simulink model "Code_Gen_Model"  (R2025a)
settings: Solver=FixedStepDiscrete  StartTime=0.0  StopTime=inf  FixedStep=t_sample  RelTol=1e-3
settings Model: Creator=FIRSTMentor  LastModifiedBy=ander
settings OptimizationCC: DefaultParameterBehavior=Inlined  StrengthReduction=on  PassReuseOutputArgsAs=Individual arguments  ZeroExternalMemoryAtStartup=off  ZeroInternalMemoryAtStartup=off  OptimizeBlockOrder=speed  OptimizationPriority=Speed  OptimizationCustomize=off  MultiThreadedLoops=on  AutoScheduleForLoops=on  EfficientTunableParamExpr=on
settings DebuggingCC: MergeDetectMultiDrivingBlocksExec=none  ParameterTunabilityLossMsg=error
settings HardwareCC: ProdBitPerPointer=32.0  ProdBitPerSizeT=32.0  ProdBitPerPtrDiffT=32.0  ProdLargestAtomicInteger=Long  ProdWordSize=32.0  ProdHWDeviceType=ARM Compatible->ARM 7
settings ModelReferenceCC: PropagateSignalLabelsOutOfModel=off
settings SFSimCC: MATLABDynamicMemAlloc=off
settings RTWCC: SystemTargetFile=ert.tlc  GenCodeOnly=on  TemplateMakefile=ert_default_tmf  Toolchain=MinGW64 | gmake (64-bit Windows)  GPUComputeCapability=3.5  Description=Embedded Coder
settings CodeAppCC: ForceParamTrailComments=on  IgnoreCustomStorageClasses=off  OperatorAnnotations=on  SimulinkDataObjDesc=on  SFDataObjDesc=on  InsertBlockDesc=on
settings ERTTargetCC: ExtModeTransport=0.0  ExtModeStaticAlloc=off  ExtModeMexFile=ext_comm  ExtModeIntrfLevel=Level1  ERTCustomFileTemplate=example_file_process.tlc  DynamicArrayContainerType=coder::array  TargetLangStandard=C99 (ISO)  SupportVariableSizeSignals=on  ParenthesesLevel=Maximum

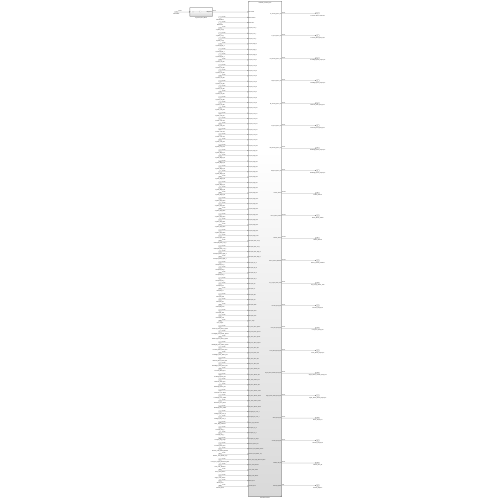
[thumbnail: Simulink's stored preview of the top-level diagram]
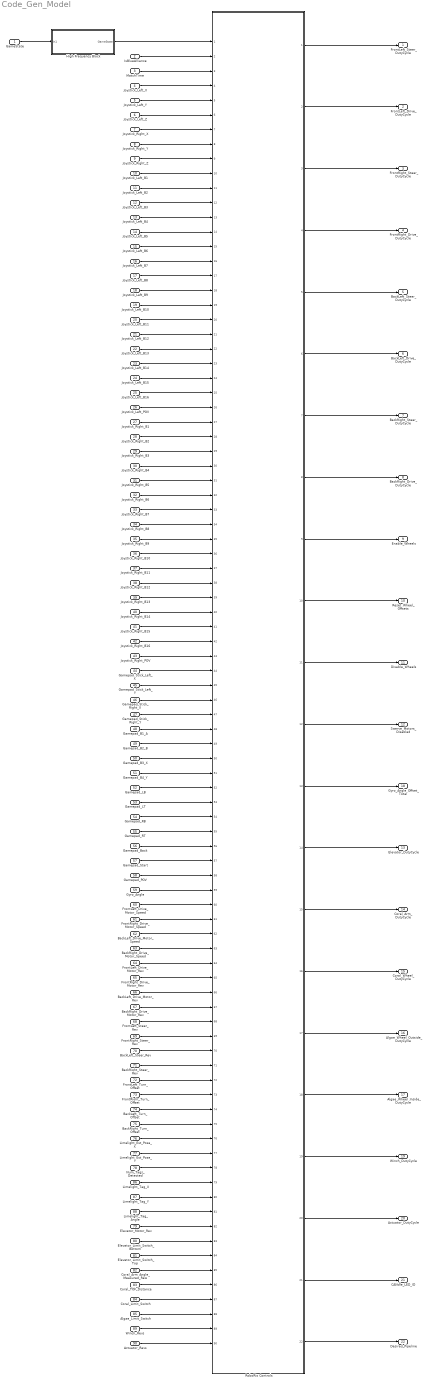
== system Code_Gen_Model ==
  GameState : Inport
  IsBlueAlliance : Inport  Port=2
  MatchTime : Inport  Port=3
  Joystick_Left_X : Inport  Port=4
  Joystick_Left_Y : Inport  Port=5
  Joystick_Left_Z : Inport  Port=6
  Joystick_Right_X : Inport  Port=7
  Joystick_Right_Y : Inport  Port=8
  Joystick_Right_Z : Inport  Port=9
  Joystick_Left_B1 : Inport  Port=10
  Joystick_Left_B2 : Inport  Port=11
  Joystick_Left_B3 : Inport  Port=12
  Joystick_Left_B4 : Inport  Port=13
  Joystick_Left_B5 : Inport  Port=14
  Joystick_Left_B6 : Inport  Port=15
  Joystick_Left_B7 : Inport  Port=16
  Joystick_Left_B8 : Inport  Port=17
  Joystick_Left_B9 : Inport  Port=18
  Joystick_Left_B10 : Inport  Port=19
  Joystick_Left_B11 : Inport  Port=20
  Joystick_Left_B12 : Inport  Port=21
  Joystick_Left_B13 : Inport  Port=22
  Joystick_Left_B14 : Inport  Port=23
  Joystick_Left_B15 : Inport  Port=24
  Joystick_Left_B16 : Inport  Port=25
  Joystick_Left_POV : Inport  Port=26
  Joystick_Right_B1 : Inport  Port=27
  Joystick_Right_B2 : Inport  Port=28
  Joystick_Right_B3 : Inport  Port=29
  Joystick_Right_B4 : Inport  Port=30
  Joystick_Right_B5 : Inport  Port=31
  Joystick_Right_B6 : Inport  Port=32
  Joystick_Right_B7 : Inport  Port=33
  Joystick_Right_B8 : Inport  Port=34
  Joystick_Right_B9 : Inport  Port=35
  Joystick_Right_B10 : Inport  Port=36
  Joystick_Right_B11 : Inport  Port=37
  Joystick_Right_B12 : Inport  Port=38
  Joystick_Right_B13 : Inport  Port=39
  Joystick_Right_B14 : Inport  Port=40
  Joystick_Right_B15 : Inport  Port=41
  Joystick_Right_B16 : Inport  Port=42
  Joystick_Right_POV : Inport  Port=43
  Gamepad_Stick_Left_X : Inport  Port=44
  Gamepad_Stick_Left_Y : Inport  Port=45
  Gamepad_Stick_Right_X : Inport  Port=46
  Gamepad_Stick_Right_Y : Inport  Port=47
  Gamepad_B1_A : Inport  Port=48
  Gamepad_B2_B : Inport  Port=49
  Gamepad_B3_X : Inport  Port=50
  Gamepad_B4_Y : Inport  Port=51
  Gamepad_LB : Inport  Port=52
  Gamepad_LT : Inport  Port=53
  Gamepad_RB : Inport  Port=54
  Gamepad_RT : Inport  Port=55
  Gamepad_Back : Inport  Port=56
  Gamepad_Start : Inport  Port=57
  Gamepad_POV : Inport  Port=58
  Gyro_Angle : Inport  Port=59
  FrontLeft_Drive_Motor_Speed : Inport  Port=60
  FrontRight_Drive_Motor_Speed : Inport  Port=61
  BackLeft_Drive_Motor_Speed : Inport  Port=62
  BackRight_Drive_Motor_Speed : Inport  Port=63
  FrontLeft_Drive_Motor_Rev : Inport  Port=64
  FrontRight_Drive_Motor_Rev : Inport  Port=65
  BackLeft_Drive_Motor_Rev : Inport  Port=66
  BackRight_Drive_Motor_Rev : Inport  Port=67
  FrontLeft_Steer_Rev : Inport  Port=68
  FrontRight_Steer_Rev : Inport  Port=69
  BackLeft_Steer_Rev : Inport  Port=70
  BackRight_Steer_Rev : Inport  Port=71
  FrontLeft_Turn_Offset : Inport  Port=72
  FrontRight_Turn_Offset : Inport  Port=73
  BackLeft_Turn_Offset : Inport  Port=74
  BackRight_Turn_Offset : Inport  Port=75
  Limelight_Est_Pose_X : Inport  Port=76
  Limelight_Est_Pose_Y : Inport  Port=77
  Num_Tags_Detected : Inport  Port=78
  Elevator_Motor_Rev : Inport  Port=79
  Elevator_Limit_Switch_Bottom : Inport  Port=80
  Elevator_Limit_Switch_Top : Inport  Port=81
  Coral_Arm_Angle_Measured_Raw : Inport  Port=82
  Coral_TOF_Distance : Inport  Port=83
  Coral_Limit_Switch : Inport  Port=84
  Algae_Limit_Switch : Inport  Port=85
  Limelight_Tag_X : Inport  Port=86
  Limelight_Tag_Y : Inport  Port=87
  Limelight_Tag_Angle : Inport  Port=88
  Winch_Revs : Inport  Port=89
  Actuator_Revs : Inport  Port=90
  High Frequency Block : Subsystem  TreatAsAtomicUnit=on  RTWFcnName=High_Frequency_Model_Step
      settings: RTWSystemCode=Nonreusable function  RTWFcnNameOpts=User specified
  RoboRio Controls : Subsystem  TreatAsAtomicUnit=on  RTWFcnName=Model_Step  ReferencedSubsystem=RoboRio_Controls_sub
      settings: RTWSystemCode=Nonreusable function  RTWFcnNameOpts=User specified
  FrontLeft_Steer_DutyCycle : Outport
  FrontLeft_Drive_DutyCycle : Outport  Port=2
  FrontRight_Steer_DutyCycle : Outport  Port=3
  FrontRight_Drive_DutyCycle : Outport  Port=4
  BackLeft_Steer_DutyCycle : Outport  Port=5
  BackLeft_Drive_DutyCycle : Outport  Port=6
  BackRight_Steer_DutyCycle : Outport  Port=7
  BackRight_Drive_DutyCycle : Outport  Port=8
  Enable_Wheels : Outport  Port=9
  Reset_Wheel_Offsets : Outport  Port=10
  Disable_Wheels : Outport  Port=11
  Swerve_Motors_Disabled : Outport  Port=12
  Elevator_DutyCycle : Outport  Port=13
  Coral_Arm_DutyCycle : Outport  Port=14
  Coral_Wheel_DutyCycle : Outport  Port=15
  Algae_Wheel_Outside_DutyCycle : Outport  Port=16
  Algae_Wheel_Inside_DutyCycle : Outport  Port=17
  Gyro_Angle_Offset_Total : Outport  Port=18
  Winch_DutyCycle : Outport  Port=19
  Actuator_DutyCycle : Outport  Port=20
  CANdle_LED_ID : Outport  Port=21
  Desired_Pipeline : Outport  Port=22
  wires:
  Joystick_Right_B10/1 -> RoboRio Controls/36
  Joystick_Right_B8/1 -> RoboRio Controls/34
  Joystick_Right_B7/1 -> RoboRio Controls/33
  Joystick_Right_B4/1 -> RoboRio Controls/30
  High Frequency Block/1(GameState) -> RoboRio Controls/1
  RoboRio Controls/8 -> BackRight_Drive_DutyCycle/1
  Gamepad_Stick_Left_X/1 -> RoboRio Controls/44
  Joystick_Right_POV/1 -> RoboRio Controls/43
  Joystick_Right_B14/1 -> RoboRio Controls/40
  Joystick_Right_B13/1 -> RoboRio Controls/39
  Joystick_Right_B3/1 -> RoboRio Controls/29
  Joystick_Right_B2/1 -> RoboRio Controls/28
  Joystick_Right_B1/1 -> RoboRio Controls/27
  Joystick_Left_POV/1 -> RoboRio Controls/26
  Limelight_Est_Pose_Y/1 -> RoboRio Controls/77
  Joystick_Left_Z/1 -> RoboRio Controls/6
  Joystick_Left_Y/1 -> RoboRio Controls/5
  Joystick_Left_X/1 -> RoboRio Controls/4
  IsBlueAlliance/1 -> RoboRio Controls/2
  Gamepad_B2_B/1 -> RoboRio Controls/49
  Joystick_Left_B1/1 -> RoboRio Controls/10
  Joystick_Right_Z/1 -> RoboRio Controls/9
  RoboRio Controls/3 -> FrontRight_Steer_DutyCycle/1
  Joystick_Right_Y/1 -> RoboRio Controls/8
  Joystick_Right_X/1 -> RoboRio Controls/7
  BackRight_Steer_Rev/1 -> RoboRio Controls/71
  Joystick_Left_B7/1 -> RoboRio Controls/16
  FrontRight_Steer_Rev/1 -> RoboRio Controls/69
  Joystick_Left_B4/1 -> RoboRio Controls/13
  Joystick_Left_B3/1 -> RoboRio Controls/12
  Joystick_Left_B2/1 -> RoboRio Controls/11
  Joystick_Left_B14/1 -> RoboRio Controls/23
  Joystick_Left_B13/1 -> RoboRio Controls/22
  Joystick_Left_B10/1 -> RoboRio Controls/19
  Joystick_Left_B8/1 -> RoboRio Controls/17
  Joystick_Left_B11/1 -> RoboRio Controls/20
  Joystick_Left_B12/1 -> RoboRio Controls/21
  Gamepad_B1_A/1 -> RoboRio Controls/48
  RoboRio Controls/1 -> FrontLeft_Steer_DutyCycle/1
  Gamepad_Stick_Right_Y/1 -> RoboRio Controls/47
  Gamepad_Stick_Right_X/1 -> RoboRio Controls/46
  Gamepad_Stick_Left_Y/1 -> RoboRio Controls/45
  Gamepad_B3_X/1 -> RoboRio Controls/50
  Gamepad_RB/1 -> RoboRio Controls/54
  Gamepad_LT/1 -> RoboRio Controls/53
  Gamepad_LB/1 -> RoboRio Controls/52
  Gamepad_B4_Y/1 -> RoboRio Controls/51
  Gyro_Angle/1 -> RoboRio Controls/59
  Gamepad_Start/1 -> RoboRio Controls/57
  Gamepad_Back/1 -> RoboRio Controls/56
  Gamepad_RT/1 -> RoboRio Controls/55
  BackRight_Drive_Motor_Speed/1 -> RoboRio Controls/63
  BackLeft_Drive_Motor_Speed/1 -> RoboRio Controls/62
  FrontRight_Drive_Motor_Speed/1 -> RoboRio Controls/61
  FrontLeft_Drive_Motor_Speed/1 -> RoboRio Controls/60
  BackLeft_Drive_Motor_Rev/1 -> RoboRio Controls/66
  FrontRight_Drive_Motor_Rev/1 -> RoboRio Controls/65
  FrontLeft_Drive_Motor_Rev/1 -> RoboRio Controls/64
  BackRight_Drive_Motor_Rev/1 -> RoboRio Controls/67
  FrontLeft_Steer_Rev/1 -> RoboRio Controls/68
  BackLeft_Steer_Rev/1 -> RoboRio Controls/70
  FrontLeft_Turn_Offset/1 -> RoboRio Controls/72
  FrontRight_Turn_Offset/1 -> RoboRio Controls/73
  BackLeft_Turn_Offset/1 -> RoboRio Controls/74
  BackRight_Turn_Offset/1 -> RoboRio Controls/75
  Limelight_Est_Pose_X/1 -> RoboRio Controls/76
  Num_Tags_Detected/1 -> RoboRio Controls/78
  RoboRio Controls/2 -> FrontLeft_Drive_DutyCycle/1
  RoboRio Controls/4 -> FrontRight_Drive_DutyCycle/1
  RoboRio Controls/6 -> BackLeft_Drive_DutyCycle/1
  RoboRio Controls/5 -> BackLeft_Steer_DutyCycle/1
  RoboRio Controls/7 -> BackRight_Steer_DutyCycle/1
  RoboRio Controls/11 -> Disable_Wheels/1
  RoboRio Controls/10 -> Reset_Wheel_Offsets/1
  RoboRio Controls/12 -> Swerve_Motors_Disabled/1
  RoboRio Controls/9 -> Enable_Wheels/1
  Joystick_Left_B5/1 -> RoboRio Controls/14
  Joystick_Left_B6/1 -> RoboRio Controls/15
  Joystick_Left_B9/1 -> RoboRio Controls/18
  Joystick_Left_B15/1 -> RoboRio Controls/24
  Joystick_Left_B16/1 -> RoboRio Controls/25
  Joystick_Right_B5/1 -> RoboRio Controls/31
  Joystick_Right_B6/1 -> RoboRio Controls/32
  Joystick_Right_B9/1 -> RoboRio Controls/35
  Joystick_Right_B11/1 -> RoboRio Controls/37
  Joystick_Right_B12/1 -> RoboRio Controls/38
  Joystick_Right_B16/1 -> RoboRio Controls/42
  Joystick_Right_B15/1 -> RoboRio Controls/41
  Gamepad_POV/1 -> RoboRio Controls/58
  RoboRio Controls/16 -> Coral_Wheel_DutyCycle/1
  RoboRio Controls/17 -> Algae_Wheel_Outside_DutyCycle/1
  RoboRio Controls/13 -> Gyro_Angle_Offset_Total/1
  Limelight_Tag_X/1 -> RoboRio Controls/79
  Limelight_Tag_Y/1 -> RoboRio Controls/80
  Limelight_Tag_Angle/1 -> RoboRio Controls/81
  RoboRio Controls/21 -> CANdle_LED_ID/1
  MatchTime/1 -> RoboRio Controls/3
  Elevator_Motor_Rev/1 -> RoboRio Controls/82
  Elevator_Limit_Switch_Bottom/1 -> RoboRio Controls/83
  Elevator_Limit_Switch_Top/1 -> RoboRio Controls/84
  Coral_Arm_Angle_Measured_Raw/1 -> RoboRio Controls/85
  Coral_TOF_Distance/1 -> RoboRio Controls/86
  Coral_Limit_Switch/1 -> RoboRio Controls/87
  Algae_Limit_Switch/1 -> RoboRio Controls/88
  Winch_Revs/1 -> RoboRio Controls/89
  Actuator_Revs/1 -> RoboRio Controls/90
  RoboRio Controls/20 -> Actuator_DutyCycle/1
  RoboRio Controls/19 -> Winch_DutyCycle/1
  RoboRio Controls/18 -> Algae_Wheel_Inside_DutyCycle/1
  RoboRio Controls/15 -> Coral_Arm_DutyCycle/1
  RoboRio Controls/14 -> Elevator_DutyCycle/1
  RoboRio Controls/22 -> Desired_Pipeline/1
  GameState/1 -> High Frequency Block/1(In1)

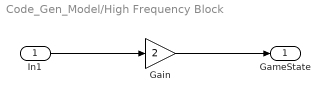
== system Code_Gen_Model/High Frequency Block ==
  In1 : Inport
  Gain : Gain  Gain=2
  GameState : Outport
  wires:
  In1/1 -> Gain/1
  Gain/1 -> GameState/1
